simulink model "FCS_MPC_6ph"  (R2022a)
settings: Solver=ode23t  StartTime=0.0  StopTime=0.1  RelTol=1e-3  AbsTol=1e-3  EnableMultiTasking=on
values from neighbouring files (symbols this model uses):
  f_c = 100000    [Params_testbench.m]
  L_d = 0.0001473    [Params_testbench.m]
  L_q = 0.0001484    [Params_testbench.m]
  L_x = 0.00005566    (= 5.566e-05)    [Params_testbench.m]
  L_y = L_x    (= 5.566e-05)    [Params_testbench.m]
  p = 5    [Params_testbench.m]
  psi_pm = 0.0048    [Params_testbench.m]
  R_ph = 0.1278    [Params_testbench.m]
  u_dc = 36.0    (= 36)    [Params_testbench.m]
libraries: nesl_utility x39, fl_lib x32, hdlsllib x25, ee_lib x12, simulink x2, spsAlphaBetaZerotodq0Lib x1
(part 3 of 4)

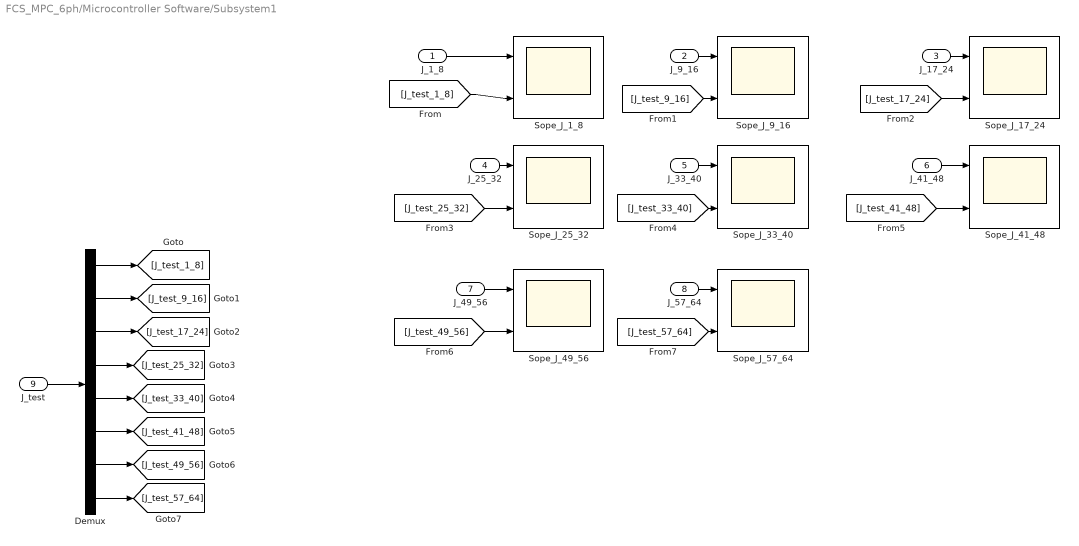
== system FCS_MPC_6ph/Microcontroller Software/Subsystem1 ==
  J_1_8 : Inport
  J_9_16 : Inport  Port=2
  J_17_24 : Inport  Port=3
  J_25_32 : Inport  Port=4
  J_33_40 : Inport  Port=5
  J_41_48 : Inport  Port=6
  J_49_56 : Inport  Port=7
  J_57_64 : Inport  Port=8
  J_test : Inport  Port=9
  Demux : Demux  Outputs=8
  Sope_J_17_24 : Scope  NumInputPorts=2
  Sope_J_1_8 : Scope  NumInputPorts=2
  Sope_J_25_32 : Scope  NumInputPorts=2
  Sope_J_33_40 : Scope  NumInputPorts=2
  Sope_J_41_48 : Scope  NumInputPorts=2
  Sope_J_49_56 : Scope  NumInputPorts=2
  Sope_J_57_64 : Scope  NumInputPorts=2
  Sope_J_9_16 : Scope  NumInputPorts=2
  wires:
  J_test/1 -> Demux/1
  J_1_8/1 -> Sope_J_1_8/1
  Demux/1 -> [J_test_1_8]
  [J_test_1_8] -> Sope_J_1_8/2
  Demux/2 -> [J_test_9_16]
  J_9_16/1 -> Sope_J_9_16/1
  J_17_24/1 -> Sope_J_17_24/1
  J_25_32/1 -> Sope_J_25_32/1
  J_33_40/1 -> Sope_J_33_40/1
  J_41_48/1 -> Sope_J_41_48/1
  J_49_56/1 -> Sope_J_49_56/1
  J_57_64/1 -> Sope_J_57_64/1
  Demux/3 -> [J_test_17_24]
  Demux/4 -> [J_test_25_32]
  Demux/5 -> [J_test_33_40]
  Demux/6 -> [J_test_41_48]
  Demux/7 -> [J_test_49_56]
  Demux/8 -> [J_test_57_64]
  [J_test_9_16] -> Sope_J_9_16/2
  [J_test_17_24] -> Sope_J_17_24/2
  [J_test_25_32] -> Sope_J_25_32/2
  [J_test_33_40] -> Sope_J_33_40/2
  [J_test_41_48] -> Sope_J_41_48/2
  [J_test_49_56] -> Sope_J_49_56/2
  [J_test_57_64] -> Sope_J_57_64/2

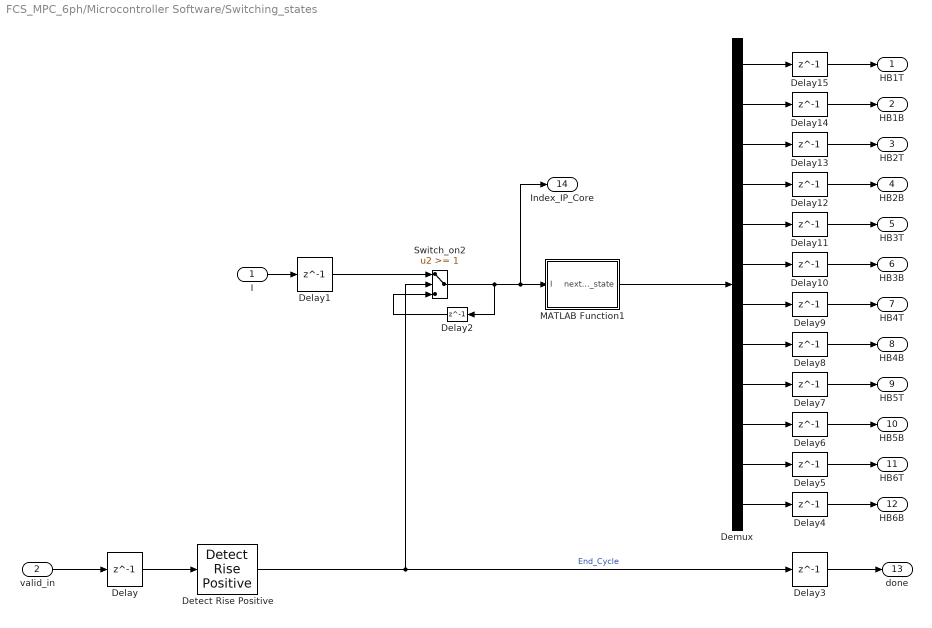
== system FCS_MPC_6ph/Microcontroller Software/Switching_states ==
  I : Inport
  valid_in : Inport  Port=2
  Delay{,1..15} (16 alike) : Delay  DelayLength=1
  Demux : Demux  Outputs=12
  Detect Rise Positive : hdlsllib/Logic and Bit Operations/Detect Rise Positive  vinit=0  OutDataTypeStr=boolean
      settings: SourceProductBaseCode=SL
  MATLAB Function1 : MATLAB Function  TreatAsAtomicUnit=on
  Switch_on2 : Switch  Threshold=1  OutDataTypeStr=Inherit: Inherit via back propagation  RndMeth=Simplest  SaturateOnIntegerOverflow=off  InputSameDT=off
  HB1T : Outport
  HB1B : Outport  Port=2
  HB2T : Outport  Port=3
  HB2B : Outport  Port=4
  HB3T : Outport  Port=5
  HB3B : Outport  Port=6
  HB4T : Outport  Port=7
  HB4B : Outport  Port=8
  HB5T : Outport  Port=9
  HB5B : Outport  Port=10
  HB6T : Outport  Port=11
  HB6B : Outport  Port=12
  done : Outport  Port=13
  Index_IP_Core : Outport  Port=14
  wires:
  Demux/4 -> Delay12/1
  I/1 -> Delay1/1
  Demux/6 -> Delay10/1
  Demux/12 -> Delay4/1
  Demux/8 -> Delay8/1
  valid_in/1 -> Delay/1
  Demux/7 -> Delay9/1
  Demux/2 -> Delay14/1
  Detect Rise Positive/1 -> Delay3/1, Switch_on2/2  "End_Cycle"
  Demux/5 -> Delay11/1
  Delay2/1 -> Switch_on2/3
  Demux/1 -> Delay15/1
  Demux/9 -> Delay7/1
  Demux/10 -> Delay6/1
  MATLAB Function1/1(next_switching_state) -> Demux/1
  Demux/3 -> Delay13/1
  Delay/1 -> Detect Rise Positive/1
  Delay1/1 -> Switch_on2/1
  Delay3/1 -> done/1
  Delay4/1 -> HB6B/1
  Demux/11 -> Delay5/1
  Delay5/1 -> HB6T/1
  Delay6/1 -> HB5B/1
  Delay7/1 -> HB5T/1
  Delay8/1 -> HB4B/1
  Delay9/1 -> HB4T/1
  Delay10/1 -> HB3B/1
  Delay11/1 -> HB3T/1
  Delay12/1 -> HB2B/1
  Delay13/1 -> HB2T/1
  Delay14/1 -> HB1B/1
  Delay15/1 -> HB1T/1
  Switch_on2/1 -> Index_IP_Core/1, MATLAB Function1/1(I), Delay2/1

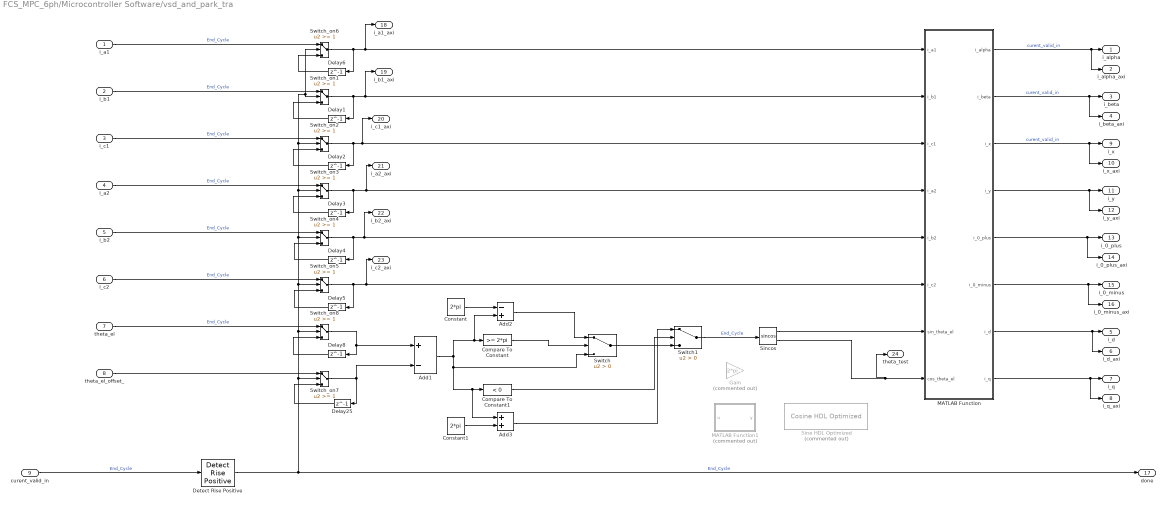
== system FCS_MPC_6ph/Microcontroller Software/vsd_and_park_tra ==
  i_a1 : Inport
  i_b1 : Inport  Port=2
  i_c1 : Inport  Port=3
  i_a2 : Inport  Port=4
  i_b2 : Inport  Port=5
  i_c2 : Inport  Port=6
  theta_el : Inport  Port=7
  theta_el_offset_ : Inport  Port=8
  curent_valid_in : Inport  Port=9
  Add1 : Sum  Inputs=+-  OutDataTypeStr=Inherit: Same as accumulator  RndMeth=Simplest
  Add2 : Sum  Inputs=-+  RndMeth=Simplest  OutDataTypeStr=Inherit: Same as first input
  Add3 : Sum  RndMeth=Simplest  OutDataTypeStr=Inherit: Same as first input
  Compare To Constant : hdlsllib/Logic and Bit Operations/Compare To Constant  relop=>=  const=2*pi  OutDataTypeStr=boolean
      settings: SourceProductBaseCode=SL
  Compare To Constant1 : hdlsllib/Logic and Bit Operations/Compare To Constant  relop=<  const=0  OutDataTypeStr=boolean
      settings: SourceProductBaseCode=SL
  Constant : Constant  Value=2*pi  OutDataTypeStr=single  SampleTime=1.0000e-08
  Constant1 : Constant  Value=2*pi  OutDataTypeStr=single  SampleTime=1.0000e-08
  Delay{1..6,8,25} (8 alike) : Delay  DelayLength=1
  Detect Rise Positive : hdlsllib/Logic and Bit Operations/Detect Rise Positive  vinit=0  OutDataTypeStr=boolean
      settings: SourceProductBaseCode=SL
  Gain : Gain  Commented=on  Gain=2*pi  OutDataTypeStr=Inherit: Same as input  ParamDataTypeStr=Inherit: Same as input
  MATLAB Function : MATLAB Function  TreatAsAtomicUnit=on  SystemSampleTime=1/100000000
  MATLAB Function1 : MATLAB Function  Commented=on  TreatAsAtomicUnit=on
  Sincos : Trigonometry  Operator=sincos
  Sine HDL Optimized : hdlsllib/Lookup Tables/Cosine HDL Optimized  Commented=on  OutputFormula=sin(2*pi*u) and cos(2*pi*u)  NumDataPoints=512  TableDataTypeStr=fixdt(1,17,11)  SimulateLUTROMDelay=off
      settings: SourceProductBaseCode=SL
  Switch : Switch  Criteria=u2 > Threshold  RndMeth=Simplest  SaturateOnIntegerOverflow=off  InputSameDT=off  OutDataTypeStr=Inherit: Same as first input
  Switch1 : Switch  Criteria=u2 > Threshold  RndMeth=Simplest  SaturateOnIntegerOverflow=off  InputSameDT=off  OutDataTypeStr=Inherit: Same as first input
  Switch_on{1..8} (8 alike) : Switch  Threshold=1  RndMeth=Simplest  SaturateOnIntegerOverflow=off  InputSameDT=off  OutDataTypeStr=Inherit: Same as first input
  i_alpha : Outport
  i_alpha_axi : Outport  Port=2
  i_beta : Outport  Port=3
  i_beta_axi : Outport  Port=4
  i_d : Outport  Port=5
  i_d_axi : Outport  Port=6
  i_q : Outport  Port=7
  i_q_axi : Outport  Port=8
  i_x : Outport  Port=9
  i_x_axi : Outport  Port=10
  i_y : Outport  Port=11
  i_y_axi : Outport  Port=12
  i_0_plus : Outport  Port=13
  i_0_plus_axi : Outport  Port=14
  i_0_minus : Outport  Port=15
  i_0_minus_axi : Outport  Port=16
  done : Outport  Port=17
  i_a1_axi : Outport  Port=18
  i_b1_axi : Outport  Port=19
  i_c1_axi : Outport  Port=20
  i_a2_axi : Outport  Port=21
  i_b2_axi : Outport  Port=22
  i_c2_axi : Outport  Port=23
  theta_test : Outport  Port=24
  wires:
  i_c2/1 -> Switch_on5/1  "End_Cycle"
  Switch_on8/1 -> Add1/1, Delay8/1
  Delay8/1 -> Switch_on8/3
  Detect Rise Positive/1 -> done/1, Switch_on7/2, Switch_on6/2, Switch_on1/2, Switch_on2/2, Switch_on3/2, Switch_on4/2, Switch_on5/2, Switch_on8/2  "End_Cycle"
  Delay4/1 -> Switch_on4/3
  Switch_on2/1 -> Delay2/1, i_c1_axi/1, MATLAB Function/3(i_c1)
  Delay1/1 -> Switch_on1/3
  Switch_on1/1 -> Delay1/1, i_b1_axi/1, MATLAB Function/2(i_b1)
  Switch_on6/1 -> i_a1_axi/1, MATLAB Function/1(i_a1), Delay6/1
  Switch_on4/1 -> Delay4/1, i_b2_axi/1, MATLAB Function/5(i_b2)
  curent_valid_in/1 -> Detect Rise Positive/1  "End_Cycle"
  Switch/1 -> Switch1/3
  Switch_on3/1 -> i_a2_axi/1, MATLAB Function/4(i_a2), Delay3/1
  Delay6/1 -> Switch_on6/3
  Constant/1 -> Add2/1
  Add1/1 -> Switch/3, Compare To Constant1/1, Add3/1, Compare To Constant/1, Add2/2
  Delay2/1 -> Switch_on2/3
  Constant1/1 -> Add3/2
  theta_el/1 -> Switch_on8/1  "End_Cycle"
  Delay3/1 -> Switch_on3/3
  i_a1/1 -> Switch_on6/1  "End_Cycle"
  i_b2/1 -> Switch_on4/1  "End_Cycle"
  Add2/1 -> Switch/1
  i_a2/1 -> Switch_on3/1  "End_Cycle"
  i_b1/1 -> Switch_on1/1  "End_Cycle"
  Delay5/1 -> Switch_on5/3
  Add3/1 -> Switch1/1
  i_c1/1 -> Switch_on2/1  "End_Cycle"
  MATLAB Function/1(i_alpha) -> i_alpha_axi/1, i_alpha/1  "curent_valid_in"
  MATLAB Function/2(i_beta) -> i_beta_axi/1, i_beta/1  "curent_valid_in"
  MATLAB Function/3(i_x) -> i_x_axi/1, i_x/1  "curent_valid_in"
  Compare To Constant/1 -> Switch/2
  Compare To Constant1/1 -> Switch1/2
  Switch_on7/1 -> Add1/2, Delay25/1
  Delay25/1 -> Switch_on7/3
  Switch1/1 -> Sincos/1  "End_Cycle"
  ? -> Sine HDL Optimized/1
  theta_el_offset_/1 -> Switch_on7/1
  MATLAB Function/8(i_q) -> i_q_axi/1, i_q/1
  MATLAB Function/7(i_d) -> i_d_axi/1, i_d/1
  MATLAB Function/6(i_0_minus) -> i_0_minus_axi/1, i_0_minus/1
  MATLAB Function/5(i_0_plus) -> i_0_plus_axi/1, i_0_plus/1
  MATLAB Function/4(i_y) -> i_y_axi/1, i_y/1
  Switch_on5/1 -> Delay5/1, i_c2_axi/1, MATLAB Function/6(i_c2)
  Sincos/1 -> MATLAB Function/7(sin_theta_el)
  Sincos/2 -> theta_test/1, MATLAB Function/8(cos_theta_el)

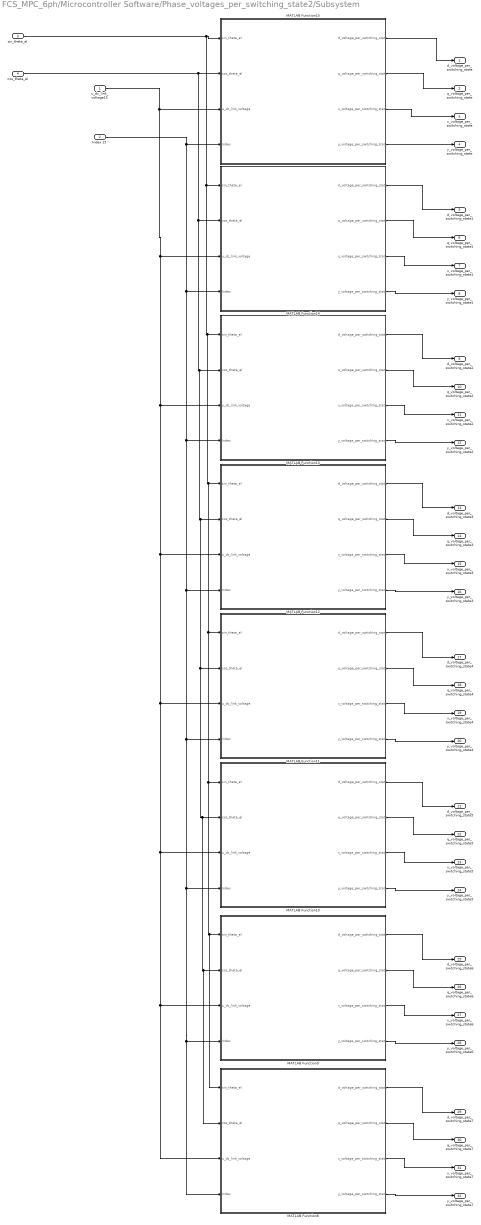
== system FCS_MPC_6ph/Microcontroller Software/Phase_voltages_per_switching_state2/Subsystem ==
  u_dc_link_voltage15 : Inport
  Index 15 : Inport  Port=2
  sin_theta_el : Inport  Port=3
  cos_theta_el : Inport  Port=4
  MATLAB Function10 : MATLAB Function  TreatAsAtomicUnit=on  SystemSampleTime=1/100000000
  MATLAB Function11 : MATLAB Function  TreatAsAtomicUnit=on  SystemSampleTime=1/100000000
  MATLAB Function12 : MATLAB Function  TreatAsAtomicUnit=on  SystemSampleTime=1/100000000
  MATLAB Function13 : MATLAB Function  TreatAsAtomicUnit=on  SystemSampleTime=1/100000000
  MATLAB Function14 : MATLAB Function  TreatAsAtomicUnit=on  SystemSampleTime=1/100000000
  MATLAB Function15 : MATLAB Function  TreatAsAtomicUnit=on  SystemSampleTime=1/100000000
  MATLAB Function8 : MATLAB Function  TreatAsAtomicUnit=on  SystemSampleTime=1/100000000
  MATLAB Function9 : MATLAB Function  TreatAsAtomicUnit=on  SystemSampleTime=1/100000000
  d_voltage_per_switching_state : Outport
  q_voltage_per_switching_state : Outport  Port=2
  x_voltage_per_switching_state : Outport  Port=3
  y_voltage_per_switching_state : Outport  Port=4
  d_voltage_per_switching_state1 : Outport  Port=5
  q_voltage_per_switching_state1 : Outport  Port=6
  x_voltage_per_switching_state1 : Outport  Port=7
  y_voltage_per_switching_state1 : Outport  Port=8
  d_voltage_per_switching_state2 : Outport  Port=9
  q_voltage_per_switching_state2 : Outport  Port=10
  x_voltage_per_switching_state2 : Outport  Port=11
  y_voltage_per_switching_state2 : Outport  Port=12
  d_voltage_per_switching_state3 : Outport  Port=13
  q_voltage_per_switching_state3 : Outport  Port=14
  x_voltage_per_switching_state3 : Outport  Port=15
  y_voltage_per_switching_state3 : Outport  Port=16
  d_voltage_per_switching_state4 : Outport  Port=17
  q_voltage_per_switching_state4 : Outport  Port=18
  x_voltage_per_switching_state4 : Outport  Port=19
  y_voltage_per_switching_state4 : Outport  Port=20
  d_voltage_per_switching_state5 : Outport  Port=21
  q_voltage_per_switching_state5 : Outport  Port=22
  x_voltage_per_switching_state5 : Outport  Port=23
  y_voltage_per_switching_state5 : Outport  Port=24
  d_voltage_per_switching_state6 : Outport  Port=25
  q_voltage_per_switching_state6 : Outport  Port=26
  x_voltage_per_switching_state6 : Outport  Port=27
  y_voltage_per_switching_state6 : Outport  Port=28
  d_voltage_per_switching_state7 : Outport  Port=29
  q_voltage_per_switching_state7 : Outport  Port=30
  x_voltage_per_switching_state7 : Outport  Port=31
  y_voltage_per_switching_state7 : Outport  Port=32
  wires:
  MATLAB Function11/4(y_voltage_per_switching_state) -> y_voltage_per_switching_state4/1
  MATLAB Function10/3(x_voltage_per_switching_state) -> x_voltage_per_switching_state5/1
  MATLAB Function8/1(d_voltage_per_switching_state) -> d_voltage_per_switching_state7/1
  MATLAB Function8/2(q_voltage_per_switching_state) -> q_voltage_per_switching_state7/1
  MATLAB Function11/1(d_voltage_per_switching_state) -> d_voltage_per_switching_state4/1
  MATLAB Function12/3(x_voltage_per_switching_state) -> x_voltage_per_switching_state3/1
  MATLAB Function15/2(q_voltage_per_switching_state) -> q_voltage_per_switching_state/1
  MATLAB Function8/3(x_voltage_per_switching_state) -> x_voltage_per_switching_state7/1
  MATLAB Function11/3(x_voltage_per_switching_state) -> x_voltage_per_switching_state4/1
  MATLAB Function10/4(y_voltage_per_switching_state) -> y_voltage_per_switching_state5/1
  MATLAB Function11/2(q_voltage_per_switching_state) -> q_voltage_per_switching_state4/1
  MATLAB Function12/1(d_voltage_per_switching_state) -> d_voltage_per_switching_state3/1
  MATLAB Function12/4(y_voltage_per_switching_state) -> y_voltage_per_switching_state3/1
  MATLAB Function13/2(q_voltage_per_switching_state) -> q_voltage_per_switching_state2/1
  MATLAB Function10/1(d_voltage_per_switching_state) -> d_voltage_per_switching_state5/1
  MATLAB Function10/2(q_voltage_per_switching_state) -> q_voltage_per_switching_state5/1
  MATLAB Function13/4(y_voltage_per_switching_state) -> y_voltage_per_switching_state2/1
  MATLAB Function8/4(y_voltage_per_switching_state) -> y_voltage_per_switching_state7/1
  MATLAB Function13/1(d_voltage_per_switching_state) -> d_voltage_per_switching_state2/1
  MATLAB Function13/3(x_voltage_per_switching_state) -> x_voltage_per_switching_state2/1
  MATLAB Function12/2(q_voltage_per_switching_state) -> q_voltage_per_switching_state3/1
  MATLAB Function15/1(d_voltage_per_switching_state) -> d_voltage_per_switching_state/1
  MATLAB Function15/4(y_voltage_per_switching_state) -> y_voltage_per_switching_state/1
  MATLAB Function15/3(x_voltage_per_switching_state) -> x_voltage_per_switching_state/1
  u_dc_link_voltage15/1 -> MATLAB Function8/3(u_dc_link_voltage), MATLAB Function9/3(u_dc_link_voltage), MATLAB Function10/3(u_dc_link_voltage), MATLAB Function11/3(u_dc_link_voltage), MATLAB Function12/3(u_dc_link_voltage), MATLAB Function13/3(u_dc_link_voltage), MATLAB Function14/3(u_dc_link_voltage), MATLAB Function15/3(u_dc_link_voltage)
  MATLAB Function14/4(y_voltage_per_switching_state) -> y_voltage_per_switching_state1/1
  MATLAB Function14/3(x_voltage_per_switching_state) -> x_voltage_per_switching_state1/1
  MATLAB Function14/1(d_voltage_per_switching_state) -> d_voltage_per_switching_state1/1
  MATLAB Function14/2(q_voltage_per_switching_state) -> q_voltage_per_switching_state1/1
  Index 15/1 -> MATLAB Function15/4(Index), MATLAB Function10/4(Index), MATLAB Function8/4(Index), MATLAB Function9/4(Index), MATLAB Function11/4(Index), MATLAB Function12/4(Index), MATLAB Function13/4(Index), MATLAB Function14/4(Index)
  MATLAB Function9/3(x_voltage_per_switching_state) -> x_voltage_per_switching_state6/1
  MATLAB Function9/2(q_voltage_per_switching_state) -> q_voltage_per_switching_state6/1
  MATLAB Function9/1(d_voltage_per_switching_state) -> d_voltage_per_switching_state6/1
  MATLAB Function9/4(y_voltage_per_switching_state) -> y_voltage_per_switching_state6/1
  sin_theta_el/1 -> MATLAB Function14/1(sin_theta_el), MATLAB Function8/1(sin_theta_el), MATLAB Function9/1(sin_theta_el), MATLAB Function10/1(sin_theta_el), MATLAB Function11/1(sin_theta_el), MATLAB Function12/1(sin_theta_el), MATLAB Function13/1(sin_theta_el), MATLAB Function15/1(sin_theta_el)
  cos_theta_el/1 -> MATLAB Function15/2(cos_theta_el), MATLAB Function8/2(cos_theta_el), MATLAB Function9/2(cos_theta_el), MATLAB Function10/2(cos_theta_el), MATLAB Function11/2(cos_theta_el), MATLAB Function12/2(cos_theta_el), MATLAB Function13/2(cos_theta_el), MATLAB Function14/2(cos_theta_el)

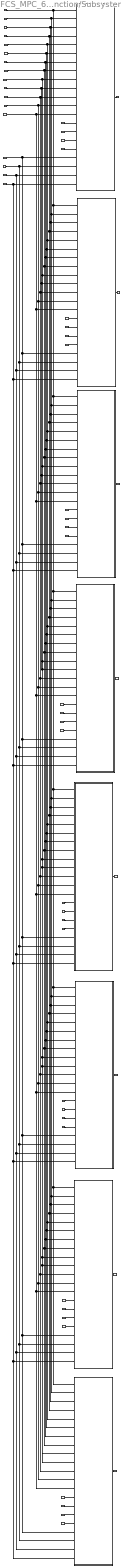
== system FCS_MPC_6ph/Microcontroller Software/Prediction_and_cost_function/Subsystem ==
  d_phase_voltage_per_switching_state : Inport
  q_phase_voltage_per_switching_state : Inport  Port=2
  x_phase_voltage_per_switching_state : Inport  Port=3
  y_phase_voltage_per_switching_state : Inport  Port=4
  d_phase_voltage_per_switching_state1 : Inport  Port=5
  q_phase_voltage_per_switching_state1 : Inport  Port=6
  x_phase_voltage_per_switching_state1 : Inport  Port=7
  y_phase_voltage_per_switching_state1 : Inport  Port=8
  d_phase_voltage_per_switching_state2 : Inport  Port=9
  q_phase_voltage_per_switching_state2 : Inport  Port=10
  x_phase_voltage_per_switching_state2 : Inport  Port=11
  y_phase_voltage_per_switching_state2 : Inport  Port=12
  d_phase_voltage_per_switching_state3 : Inport  Port=13
  q_phase_voltage_per_switching_state3 : Inport  Port=14
  x_phase_voltage_per_switching_state3 : Inport  Port=15
  y_phase_voltage_per_switching_state3 : Inport  Port=16
  d_phase_voltage_per_switching_state4 : Inport  Port=17
  q_phase_voltage_per_switching_state4 : Inport  Port=18
  x_phase_voltage_per_switching_state4 : Inport  Port=19
  y_phase_voltage_per_switching_state4 : Inport  Port=20
  d_phase_voltage_per_switching_state5 : Inport  Port=21
  q_phase_voltage_per_switching_state5 : Inport  Port=22
  x_phase_voltage_per_switching_state5 : Inport  Port=23
  y_phase_voltage_per_switching_state5 : Inport  Port=24
  d_phase_voltage_per_switching_state6 : Inport  Port=25
  q_phase_voltage_per_switching_state6 : Inport  Port=26
  x_phase_voltage_per_switching_state6 : Inport  Port=27
  y_phase_voltage_per_switching_state6 : Inport  Port=28
  d_phase_voltage_per_switching_state7 : Inport  Port=29
  q_phase_voltage_per_switching_state7 : Inport  Port=30
  x_phase_voltage_per_switching_state7 : Inport  Port=31
  y_phase_voltage_per_switching_state7 : Inport  Port=32
  SampleTime_div_Ld15 : Inport  Port=33
  SampleTime_div_Lq15 : Inport  Port=34
  SampleTime_div_Lx15 : Inport  Port=35
  SampleTime_div_Ly15 : Inport  Port=36
  id_k_16 : Inport  Port=37
  iq_k_16 : Inport  Port=38
  ix_k_16 : Inport  Port=39
  iy_k_16 : Inport  Port=40
  Rs15 : Inport  Port=41
  omega_el15 : Inport  Port=42
  Lq15 : Inport  Port=43
  Ld15 : Inport  Port=44
  psiPM15 : Inport  Port=45
  id_ref15 : Inport  Port=46
  iq_ref15 : Inport  Port=47
  ix_ref15 : Inport  Port=48
  iy_ref15 : Inport  Port=49
  MATLAB Function10 : MATLAB Function  TreatAsAtomicUnit=on  SystemSampleTime=1/100000000
  MATLAB Function11 : MATLAB Function  TreatAsAtomicUnit=on  SystemSampleTime=1/100000000
  MATLAB Function12 : MATLAB Function  TreatAsAtomicUnit=on  SystemSampleTime=1/100000000
  MATLAB Function13 : MATLAB Function  TreatAsAtomicUnit=on  SystemSampleTime=1/100000000
  MATLAB Function14 : MATLAB Function  TreatAsAtomicUnit=on  SystemSampleTime=1/100000000
  MATLAB Function15 : MATLAB Function  TreatAsAtomicUnit=on  SystemSampleTime=1/100000000
  MATLAB Function8 : MATLAB Function  TreatAsAtomicUnit=on  SystemSampleTime=1/100000000
  MATLAB Function9 : MATLAB Function  TreatAsAtomicUnit=on  SystemSampleTime=1/100000000
  J : Outport
  J1 : Outport  Port=2
  J2 : Outport  Port=3
  J3 : Outport  Port=4
  J4 : Outport  Port=5
  J5 : Outport  Port=6
  J6 : Outport  Port=7
  J7 : Outport  Port=8
  wires:
  q_phase_voltage_per_switching_state1/1 -> MATLAB Function14/15(q_phase_voltage_per_switching_state)
  SampleTime_div_Ld15/1 -> MATLAB Function8/1(SampleTime_div_Ld), MATLAB Function9/1(SampleTime_div_Ld), MATLAB Function10/1(SampleTime_div_Ld), MATLAB Function11/1(SampleTime_div_Ld), MATLAB Function12/1(SampleTime_div_Ld), MATLAB Function13/1(SampleTime_div_Ld), MATLAB Function14/1(SampleTime_div_Ld), MATLAB Function15/1(SampleTime_div_Ld)
  Rs15/1 -> MATLAB Function8/9(Rs), MATLAB Function9/9(Rs), MATLAB Function10/9(Rs), MATLAB Function11/9(Rs), MATLAB Function12/9(Rs), MATLAB Function13/9(Rs), MATLAB Function14/9(Rs), MATLAB Function15/9(Rs)
  y_phase_voltage_per_switching_state/1 -> MATLAB Function15/17(y_phase_voltage_per_switching_state)
  Lq15/1 -> MATLAB Function8/11(Lq), MATLAB Function9/11(Lq), MATLAB Function10/11(Lq), MATLAB Function11/11(Lq), MATLAB Function12/11(Lq), MATLAB Function13/11(Lq), MATLAB Function14/11(Lq), MATLAB Function15/11(Lq)
  MATLAB Function11/1(J) -> J4/1
  y_phase_voltage_per_switching_state2/1 -> MATLAB Function13/17(y_phase_voltage_per_switching_state)
  d_phase_voltage_per_switching_state1/1 -> MATLAB Function14/14(d_phase_voltage_per_switching_state)
  x_phase_voltage_per_switching_state1/1 -> MATLAB Function14/16(x_phase_voltage_per_switching_state)
  y_phase_voltage_per_switching_state7/1 -> MATLAB Function8/17(y_phase_voltage_per_switching_state)
  iy_ref15/1 -> MATLAB Function8/21(iy_ref), MATLAB Function9/21(iy_ref), MATLAB Function10/21(iy_ref), MATLAB Function11/21(iy_ref), MATLAB Function12/21(iy_ref), MATLAB Function13/21(iy_ref), MATLAB Function14/21(iy_ref), MATLAB Function15/21(iy_ref)
  omega_el15/1 -> MATLAB Function8/10(omega_el), MATLAB Function9/10(omega_el), MATLAB Function10/10(omega_el), MATLAB Function11/10(omega_el), MATLAB Function12/10(omega_el), MATLAB Function13/10(omega_el), MATLAB Function14/10(omega_el), MATLAB Function15/10(omega_el)
  psiPM15/1 -> MATLAB Function8/13(psiPM), MATLAB Function9/13(psiPM), MATLAB Function10/13(psiPM), MATLAB Function11/13(psiPM), MATLAB Function12/13(psiPM), MATLAB Function13/13(psiPM), MATLAB Function14/13(psiPM), MATLAB Function15/13(psiPM)
  d_phase_voltage_per_switching_state3/1 -> MATLAB Function12/14(d_phase_voltage_per_switching_state)
  d_phase_voltage_per_switching_state6/1 -> MATLAB Function9/14(d_phase_voltage_per_switching_state)
  d_phase_voltage_per_switching_state/1 -> MATLAB Function15/14(d_phase_voltage_per_switching_state)
  x_phase_voltage_per_switching_state3/1 -> MATLAB Function12/16(x_phase_voltage_per_switching_state)
  d_phase_voltage_per_switching_state2/1 -> MATLAB Function13/14(d_phase_voltage_per_switching_state)
  x_phase_voltage_per_switching_state4/1 -> MATLAB Function11/16(x_phase_voltage_per_switching_state)
  y_phase_voltage_per_switching_state1/1 -> MATLAB Function14/17(y_phase_voltage_per_switching_state)
  MATLAB Function14/1(J) -> J1/1
  MATLAB Function8/1(J) -> J7/1
  q_phase_voltage_per_switching_state2/1 -> MATLAB Function13/15(q_phase_voltage_per_switching_state)
  x_phase_voltage_per_switching_state2/1 -> MATLAB Function13/16(x_phase_voltage_per_switching_state)
  MATLAB Function13/1(J) -> J2/1
  y_phase_voltage_per_switching_state4/1 -> MATLAB Function11/17(y_phase_voltage_per_switching_state)
  x_phase_voltage_per_switching_state/1 -> MATLAB Function15/16(x_phase_voltage_per_switching_state)
  q_phase_voltage_per_switching_state5/1 -> MATLAB Function10/15(q_phase_voltage_per_switching_state)
  d_phase_voltage_per_switching_state7/1 -> MATLAB Function8/14(d_phase_voltage_per_switching_state)
  d_phase_voltage_per_switching_state4/1 -> MATLAB Function11/14(d_phase_voltage_per_switching_state)
  q_phase_voltage_per_switching_state4/1 -> MATLAB Function11/15(q_phase_voltage_per_switching_state)
  x_phase_voltage_per_switching_state5/1 -> MATLAB Function10/16(x_phase_voltage_per_switching_state)
  SampleTime_div_Lx15/1 -> MATLAB Function8/3(SampleTime_div_Lx), MATLAB Function9/3(SampleTime_div_Lx), MATLAB Function10/3(SampleTime_div_Lx), MATLAB Function11/3(SampleTime_div_Lx), MATLAB Function12/3(SampleTime_div_Lx), MATLAB Function13/3(SampleTime_div_Lx), MATLAB Function14/3(SampleTime_div_Lx), MATLAB Function15/3(SampleTime_div_Lx)
  SampleTime_div_Ly15/1 -> MATLAB Function8/4(SampleTime_div_Ly), MATLAB Function9/4(SampleTime_div_Ly), MATLAB Function10/4(SampleTime_div_Ly), MATLAB Function11/4(SampleTime_div_Ly), MATLAB Function12/4(SampleTime_div_Ly), MATLAB Function13/4(SampleTime_div_Ly), MATLAB Function14/4(SampleTime_div_Ly), MATLAB Function15/4(SampleTime_div_Ly)
  SampleTime_div_Lq15/1 -> MATLAB Function8/2(SampleTime_div_Lq), MATLAB Function9/2(SampleTime_div_Lq), MATLAB Function10/2(SampleTime_div_Lq), MATLAB Function11/2(SampleTime_div_Lq), MATLAB Function12/2(SampleTime_div_Lq), MATLAB Function13/2(SampleTime_div_Lq), MATLAB Function14/2(SampleTime_div_Lq), MATLAB Function15/2(SampleTime_div_Lq)
  x_phase_voltage_per_switching_state7/1 -> MATLAB Function8/16(x_phase_voltage_per_switching_state)
  q_phase_voltage_per_switching_state/1 -> MATLAB Function15/15(q_phase_voltage_per_switching_state)
  MATLAB Function15/1(J) -> J/1
  d_phase_voltage_per_switching_state5/1 -> MATLAB Function10/14(d_phase_voltage_per_switching_state)
  MATLAB Function10/1(J) -> J5/1
  y_phase_voltage_per_switching_state5/1 -> MATLAB Function10/17(y_phase_voltage_per_switching_state)
  q_phase_voltage_per_switching_state6/1 -> MATLAB Function9/15(q_phase_voltage_per_switching_state)
  y_phase_voltage_per_switching_state6/1 -> MATLAB Function9/17(y_phase_voltage_per_switching_state)
  x_phase_voltage_per_switching_state6/1 -> MATLAB Function9/16(x_phase_voltage_per_switching_state)
  MATLAB Function9/1(J) -> J6/1
  MATLAB Function12/1(J) -> J3/1
  q_phase_voltage_per_switching_state7/1 -> MATLAB Function8/15(q_phase_voltage_per_switching_state)
  y_phase_voltage_per_switching_state3/1 -> MATLAB Function12/17(y_phase_voltage_per_switching_state)
  q_phase_voltage_per_switching_state3/1 -> MATLAB Function12/15(q_phase_voltage_per_switching_state)
  ix_ref15/1 -> MATLAB Function8/20(ix_ref), MATLAB Function9/20(ix_ref), MATLAB Function10/20(ix_ref), MATLAB Function11/20(ix_ref), MATLAB Function12/20(ix_ref), MATLAB Function13/20(ix_ref), MATLAB Function14/20(ix_ref), MATLAB Function15/20(ix_ref)
  iq_ref15/1 -> MATLAB Function8/19(iq_ref), MATLAB Function9/19(iq_ref), MATLAB Function10/19(iq_ref), MATLAB Function11/19(iq_ref), MATLAB Function12/19(iq_ref), MATLAB Function13/19(iq_ref), MATLAB Function14/19(iq_ref), MATLAB Function15/19(iq_ref)
  id_ref15/1 -> MATLAB Function8/18(id_ref), MATLAB Function9/18(id_ref), MATLAB Function10/18(id_ref), MATLAB Function11/18(id_ref), MATLAB Function12/18(id_ref), MATLAB Function13/18(id_ref), MATLAB Function14/18(id_ref), MATLAB Function15/18(id_ref)
  Ld15/1 -> MATLAB Function8/12(Ld), MATLAB Function9/12(Ld), MATLAB Function10/12(Ld), MATLAB Function11/12(Ld), MATLAB Function12/12(Ld), MATLAB Function13/12(Ld), MATLAB Function14/12(Ld), MATLAB Function15/12(Ld)
  iy_k_16/1 -> MATLAB Function8/8(iy_k_1), MATLAB Function9/8(iy_k_1), MATLAB Function10/8(iy_k_1), MATLAB Function11/8(iy_k_1), MATLAB Function12/8(iy_k_1), MATLAB Function13/8(iy_k_1), MATLAB Function14/8(iy_k_1), MATLAB Function15/8(iy_k_1)
  ix_k_16/1 -> MATLAB Function8/7(ix_k_1), MATLAB Function9/7(ix_k_1), MATLAB Function10/7(ix_k_1), MATLAB Function11/7(ix_k_1), MATLAB Function12/7(ix_k_1), MATLAB Function13/7(ix_k_1), MATLAB Function14/7(ix_k_1), MATLAB Function15/7(ix_k_1)
  iq_k_16/1 -> MATLAB Function8/6(iq_k_1), MATLAB Function9/6(iq_k_1), MATLAB Function10/6(iq_k_1), MATLAB Function11/6(iq_k_1), MATLAB Function12/6(iq_k_1), MATLAB Function13/6(iq_k_1), MATLAB Function14/6(iq_k_1), MATLAB Function15/6(iq_k_1)
  id_k_16/1 -> MATLAB Function8/5(id_k_1), MATLAB Function9/5(id_k_1), MATLAB Function10/5(id_k_1), MATLAB Function11/5(id_k_1), MATLAB Function12/5(id_k_1), MATLAB Function13/5(id_k_1), MATLAB Function14/5(id_k_1), MATLAB Function15/5(id_k_1)

== matlab function FCS_MPC_6ph/Microcontroller Software/Phase_voltages_per_switching_state2/MATLAB Function1 ==
  settings: fimath=fimath('RoundingMethod', 'Floor','OverflowAction', 'Wrap','ProductMode', 'FullPrecision', 'SumMode', 'FullPrecision')
  data: u input; y output
function y = fcn(u)

    y = fi(u*(1/(2*pi)));

end

== matlab function FCS_MPC_6ph/Microcontroller Software/Switching_states/MATLAB Function1 ==
  data: I input; next_switching_state output
function next_switching_state = fcn(I)

    % Possible switching states of the 6-Phase 2-level inverter
    possible_swichting_states = [0	1	0	1	0	1	0	1	0	1	0	1;
                                1	0	0	1	0	1	0	1	0	1	0	1;
                                0	1	1	0	0	1	0	1	0	1	0	1;
                                1	0	1	0	0	1	0	1	0	1	0	1;
                                0	1	0	1	1	0	0	1	0	1	0	1;
                                1	0	0	1	1	0	0	1	0	1	0	1;
                                0	1	1	0	1	0	0	1	0	1	0	1;
                                1	0	1	0	1	0	0	1	0	1	0	1;
                                0	1	0	1	0	1	1	0	0	1	0	1;
                                1	0	0	1	0	1	1	0	0	1	0	1;
                                0	1	1	0	0	1	1	0	0	1	0	1;
                                1	0	1	0	0	1	1	0	0	1	0	1;
                                0	1	0	1	1	0	1	0	0	1	0	1;
                                1	0	0	1	1	0	1	0	0	1	0	1;
                                0	1	1	0	1	0	1	0	0	1	0	1;
                                1	0	1	0	1	0	1	0	0	1	0	1;
                                0	1	0	1	0	1	0	1	1	0	0	1;
                                1	0	0	1	0	1	0	1	1	0	0	1;
                                0	1	1	0	0	1	0	1	1	0	0	1;
                                1	0	1	0	0	1	0	1	1	0	0	1;
                                0	1	0	1	1	0	0	1	1	0	0	1;
                                1	0	0	1	1	0	0	1	1	0	0	1;
                                0	1	1	0	1	0	0	1	1	0	0	1;
                                1	0	1	0	1	0	0	1	1	0	0	1;
                                0	1	0	1	0	1	1	0	1	0	0	1;
                                1	0	0	1	0	1	1	0	1	0	0	1;
                                0	1	1	0	0	1	1	0	1	0	0	1;
                                1	0	1	0	0	1	1	0	1	0	0	1;
                                0	1	0	1	1	0	1	0	1	0	0	1;
                                1	0	0	1	1	0	1	0	1	0	0	1;
                                0	1	1	0	1	0	1	0	1	0	0	1;
                                1	0	1	0	1	0	1	0	1	0	0	1;
                                0	1	0	1	0	1	0	1	0	1	1	0;
                                1	0	0	1	0	1	0	1	0	1	1	0;
                                0	1	1	0	0	1	0	1	0	1	1	0;
                                1	0	1	0	0	1	0	1	0	1	1	0;
                                0	1	0	1	1	0	0	1	0	1	1	0;
                                1	0	0	1	1	0	0	1	0	1	1	0;
                                0	1	1	0	1	0	0	1	0	1	1	0;
                                1	0	1	0	1	0	0	1	0	1	1	0;
                                0	1	0	1	0	1	1	0	0	1	1	0;
                                1	0	0	1	0	1	1	0	0	1	1	0;
                                0	1	1	0	0	1	1	0	0	1	1	0;
                                1	0	1	0	0	1	1	0	0	1	1	0;
                                0	1	0	1	1	0	1	0	0	1	1	0;
                                1	0	0	1	1	0	1	0	0	1	1	0;
                                0	1	1	0	1	0	1	0	0	1	1	0;
                                1	0	1	0	1	0	1	0	0	1	1	0;
                                0	1	0	1	0	1	0	1	1	0	1	0;
                                1	0	0	1	0	1	0	1	1	0	1	0;
                                0	1	1	0	0	1	0	1	1	0	1	0;
                                1	0	1	0	0	1	0	1	1	0	1	0;
                                0	1	0	1	1	0	0	1	1	0	1	0;
                                1	0	0	1	1	0	0	1	1	0	1	0;
                                0	1	1	0	1	0	0	1	1	0	1	0;
                                1	0	1	0	1	0	0	1	1	0	1	0;
                                0	1	0	1	0	1	1	0	1	0	1	0;
                                1	0	0	1	0	1	1	0	1	0	1	0;
                                0	1	1	0	0	1	1	0	1	0	1	0;
                                1	0	1	0	0	1	1	0	1	0	1	0;
                                0	1	0	1	1	0	1	0	1	0	1	0;
                                1	0	0	1	1	0	1	0	1	0	1	0;
                                0	1	1	0	1	0	1	0	1	0	1	0;
                                1	0	1	0	1	0	1	0	1	0	1	0];

    % Initial condition
    if I==0
        I=int32(1);
    end

    % Output switching state
    next_switching_state=boolean(possible_swichting_states(I,:))';

end

== matlab function FCS_MPC_6ph/6ph_PMSM_30deg_VSD1 ==
  data: u1 input; y1 output; u2 input; u3 input; u4 input; u5 input; u6 input; y2 output; y3 output; y4 output; y5 output; y6 output; k6 input; c6 input
function [y1,y2,y3,y4,y5,y6] = VSD_asymm_30(u1,u2,u3,u4,u5,u6,k6,c6)

A =single([0 0 0 0 0 0]');

A =    k6*[1    -0.5        -0.5        sqrt(3)/2   -sqrt(3)/2  0 ;
           0    sqrt(3)/2   -sqrt(3)/2  0.5         0.5         -1;
           1    -0.5        -0.5        -sqrt(3)/2  sqrt(3)/2   0 ;
           0    -sqrt(3)/2  sqrt(3)/2   0.5         0.5         -1;
           c6   c6          c6          0           0           0 ;
           0    0           0           c6          c6          c6] * [u1 u2 u3 u4 u5 u6]';

y1 =single(A(1));
y2 =single(A(2));
y3 =single(A(3));
y4 =single(A(4));
y5 =single(A(5));
y6 =single(A(6));

== matlab function FCS_MPC_6ph/Microcontroller Software/Prediction_and_cost_function/Subsystem/MATLAB Function8 ==
  data: SampleTime_div_Ld input; J output; SampleTime_div_Lq input; SampleTime_div_Lx input; SampleTime_div_Ly input; id_k_1 input; iq_k_1 input; ix_k_1 input; iy_k_1 input; Rs input; omega_el input; Lq input; Ld input; psiPM input; d_phase_voltage_per_switching_state input; q_phase_voltage_per_switching_state input; x_phase_voltage_per_switching_state input; y_phase_voltage_per_switching_state input; id_ref input; iq_ref input; ix_ref input; iy_ref input
function J = fcn(SampleTime_div_Ld, SampleTime_div_Lq, SampleTime_div_Lx, SampleTime_div_Ly, id_k_1, iq_k_1, ix_k_1, iy_k_1, Rs, omega_el, Lq, Ld, psiPM, d_phase_voltage_per_switching_state, q_phase_voltage_per_switching_state, x_phase_voltage_per_switching_state, y_phase_voltage_per_switching_state, id_ref, iq_ref, ix_ref, iy_ref)
     
        % Prediction of the d-, q-, x-, y-currents of the 6-Phase-PMSM with the finite control set 
        id_k_2 = single(SampleTime_div_Ld*(d_phase_voltage_per_switching_state-id_k_1*Rs+omega_el*Lq*iq_k_1)+id_k_1);
        iq_k_2 = single(SampleTime_div_Lq*(q_phase_voltage_per_switching_state-iq_k_1*Rs-omega_el*(psiPM+id_k_1*Ld))+iq_k_1);
        ix_k_2 = single(SampleTime_div_Lx*(x_phase_voltage_per_switching_state-ix_k_1*Rs)+ix_k_1);
        iy_k_2 = single(SampleTime_div_Ly*(y_phase_voltage_per_switching_state-iy_k_1*Rs)+iy_k_1);
        
        % Calculation of the cost function
        J = single((id_ref-id_k_2)^2+(iq_ref-iq_k_2)^2+(ix_ref-ix_k_2)^2+(iy_ref-iy_k_2)^2);

end

== matlab function FCS_MPC_6ph/Microcontroller Software/Prediction_and_cost_function/Subsystem/MATLAB Function9 ==
  data: SampleTime_div_Ld input; J output; SampleTime_div_Lq input; SampleTime_div_Lx input; SampleTime_div_Ly input; id_k_1 input; iq_k_1 input; ix_k_1 input; iy_k_1 input; Rs input; omega_el input; Lq input; Ld input; psiPM input; d_phase_voltage_per_switching_state input; q_phase_voltage_per_switching_state input; x_phase_voltage_per_switching_state input; y_phase_voltage_per_switching_state input; id_ref input; iq_ref input; ix_ref input; iy_ref input
function J = fcn(SampleTime_div_Ld, SampleTime_div_Lq, SampleTime_div_Lx, SampleTime_div_Ly, id_k_1, iq_k_1, ix_k_1, iy_k_1, Rs, omega_el, Lq, Ld, psiPM, d_phase_voltage_per_switching_state, q_phase_voltage_per_switching_state, x_phase_voltage_per_switching_state, y_phase_voltage_per_switching_state, id_ref, iq_ref, ix_ref, iy_ref)
     
        % Prediction of the d-, q-, x-, y-currents of the 6-Phase-PMSM with the finite control set 
        id_k_2 = single(SampleTime_div_Ld*(d_phase_voltage_per_switching_state-id_k_1*Rs+omega_el*Lq*iq_k_1)+id_k_1);
        iq_k_2 = single(SampleTime_div_Lq*(q_phase_voltage_per_switching_state-iq_k_1*Rs-omega_el*(psiPM+id_k_1*Ld))+iq_k_1);
        ix_k_2 = single(SampleTime_div_Lx*(x_phase_voltage_per_switching_state-ix_k_1*Rs)+ix_k_1);
        iy_k_2 = single(SampleTime_div_Ly*(y_phase_voltage_per_switching_state-iy_k_1*Rs)+iy_k_1);
        
        % Calculation of the cost function
        J = single((id_ref-id_k_2)^2+(iq_ref-iq_k_2)^2+(ix_ref-ix_k_2)^2+(iy_ref-iy_k_2)^2);

end

== matlab function FCS_MPC_6ph/Microcontroller Software/Prediction_and_cost_function/Subsystem/MATLAB Function10 ==
  data: SampleTime_div_Ld input; J output; SampleTime_div_Lq input; SampleTime_div_Lx input; SampleTime_div_Ly input; id_k_1 input; iq_k_1 input; ix_k_1 input; iy_k_1 input; Rs input; omega_el input; Lq input; Ld input; psiPM input; d_phase_voltage_per_switching_state input; q_phase_voltage_per_switching_state input; x_phase_voltage_per_switching_state input; y_phase_voltage_per_switching_state input; id_ref input; iq_ref input; ix_ref input; iy_ref input
function J = fcn(SampleTime_div_Ld, SampleTime_div_Lq, SampleTime_div_Lx, SampleTime_div_Ly, id_k_1, iq_k_1, ix_k_1, iy_k_1, Rs, omega_el, Lq, Ld, psiPM, d_phase_voltage_per_switching_state, q_phase_voltage_per_switching_state, x_phase_voltage_per_switching_state, y_phase_voltage_per_switching_state, id_ref, iq_ref, ix_ref, iy_ref)
     
        % Prediction of the d-, q-, x-, y-currents of the 6-Phase-PMSM with the finite control set 
        id_k_2 = single(SampleTime_div_Ld*(d_phase_voltage_per_switching_state-id_k_1*Rs+omega_el*Lq*iq_k_1)+id_k_1);
        iq_k_2 = single(SampleTime_div_Lq*(q_phase_voltage_per_switching_state-iq_k_1*Rs-omega_el*(psiPM+id_k_1*Ld))+iq_k_1);
        ix_k_2 = single(SampleTime_div_Lx*(x_phase_voltage_per_switching_state-ix_k_1*Rs)+ix_k_1);
        iy_k_2 = single(SampleTime_div_Ly*(y_phase_voltage_per_switching_state-iy_k_1*Rs)+iy_k_1);
        
        % Calculation of the cost function
        J = single((id_ref-id_k_2)^2+(iq_ref-iq_k_2)^2+(ix_ref-ix_k_2)^2+(iy_ref-iy_k_2)^2);

end

== matlab function FCS_MPC_6ph/Microcontroller Software/Prediction_and_cost_function/Subsystem/MATLAB Function11 ==
  data: SampleTime_div_Ld input; J output; SampleTime_div_Lq input; SampleTime_div_Lx input; SampleTime_div_Ly input; id_k_1 input; iq_k_1 input; ix_k_1 input; iy_k_1 input; Rs input; omega_el input; Lq input; Ld input; psiPM input; d_phase_voltage_per_switching_state input; q_phase_voltage_per_switching_state input; x_phase_voltage_per_switching_state input; y_phase_voltage_per_switching_state input; id_ref input; iq_ref input; ix_ref input; iy_ref input
function J = fcn(SampleTime_div_Ld, SampleTime_div_Lq, SampleTime_div_Lx, SampleTime_div_Ly, id_k_1, iq_k_1, ix_k_1, iy_k_1, Rs, omega_el, Lq, Ld, psiPM, d_phase_voltage_per_switching_state, q_phase_voltage_per_switching_state, x_phase_voltage_per_switching_state, y_phase_voltage_per_switching_state, id_ref, iq_ref, ix_ref, iy_ref)
     
        % Prediction of the d-, q-, x-, y-currents of the 6-Phase-PMSM with the finite control set 
        id_k_2 = single(SampleTime_div_Ld*(d_phase_voltage_per_switching_state-id_k_1*Rs+omega_el*Lq*iq_k_1)+id_k_1);
        iq_k_2 = single(SampleTime_div_Lq*(q_phase_voltage_per_switching_state-iq_k_1*Rs-omega_el*(psiPM+id_k_1*Ld))+iq_k_1);
        ix_k_2 = single(SampleTime_div_Lx*(x_phase_voltage_per_switching_state-ix_k_1*Rs)+ix_k_1);
        iy_k_2 = single(SampleTime_div_Ly*(y_phase_voltage_per_switching_state-iy_k_1*Rs)+iy_k_1);
        
        % Calculation of the cost function
        J = single((id_ref-id_k_2)^2+(iq_ref-iq_k_2)^2+(ix_ref-ix_k_2)^2+(iy_ref-iy_k_2)^2);

end

== matlab function FCS_MPC_6ph/Microcontroller Software/Prediction_and_cost_function/Subsystem/MATLAB Function12 ==
  data: SampleTime_div_Ld input; J output; SampleTime_div_Lq input; SampleTime_div_Lx input; SampleTime_div_Ly input; id_k_1 input; iq_k_1 input; ix_k_1 input; iy_k_1 input; Rs input; omega_el input; Lq input; Ld input; psiPM input; d_phase_voltage_per_switching_state input; q_phase_voltage_per_switching_state input; x_phase_voltage_per_switching_state input; y_phase_voltage_per_switching_state input; id_ref input; iq_ref input; ix_ref input; iy_ref input
function J = fcn(SampleTime_div_Ld, SampleTime_div_Lq, SampleTime_div_Lx, SampleTime_div_Ly, id_k_1, iq_k_1, ix_k_1, iy_k_1, Rs, omega_el, Lq, Ld, psiPM, d_phase_voltage_per_switching_state, q_phase_voltage_per_switching_state, x_phase_voltage_per_switching_state, y_phase_voltage_per_switching_state, id_ref, iq_ref, ix_ref, iy_ref)
     
        % Prediction of the d-, q-, x-, y-currents of the 6-Phase-PMSM with the finite control set 
        id_k_2 = single(SampleTime_div_Ld*(d_phase_voltage_per_switching_state-id_k_1*Rs+omega_el*Lq*iq_k_1)+id_k_1);
        iq_k_2 = single(SampleTime_div_Lq*(q_phase_voltage_per_switching_state-iq_k_1*Rs-omega_el*(psiPM+id_k_1*Ld))+iq_k_1);
        ix_k_2 = single(SampleTime_div_Lx*(x_phase_voltage_per_switching_state-ix_k_1*Rs)+ix_k_1);
        iy_k_2 = single(SampleTime_div_Ly*(y_phase_voltage_per_switching_state-iy_k_1*Rs)+iy_k_1);
        
        % Calculation of the cost function
        J = single((id_ref-id_k_2)^2+(iq_ref-iq_k_2)^2+(ix_ref-ix_k_2)^2+(iy_ref-iy_k_2)^2);

end

== matlab function FCS_MPC_6ph/Microcontroller Software/Prediction_and_cost_function/Subsystem/MATLAB Function13 ==
  data: SampleTime_div_Ld input; J output; SampleTime_div_Lq input; SampleTime_div_Lx input; SampleTime_div_Ly input; id_k_1 input; iq_k_1 input; ix_k_1 input; iy_k_1 input; Rs input; omega_el input; Lq input; Ld input; psiPM input; d_phase_voltage_per_switching_state input; q_phase_voltage_per_switching_state input; x_phase_voltage_per_switching_state input; y_phase_voltage_per_switching_state input; id_ref input; iq_ref input; ix_ref input; iy_ref input
function J = fcn(SampleTime_div_Ld, SampleTime_div_Lq, SampleTime_div_Lx, SampleTime_div_Ly, id_k_1, iq_k_1, ix_k_1, iy_k_1, Rs, omega_el, Lq, Ld, psiPM, d_phase_voltage_per_switching_state, q_phase_voltage_per_switching_state, x_phase_voltage_per_switching_state, y_phase_voltage_per_switching_state, id_ref, iq_ref, ix_ref, iy_ref)
     
        % Prediction of the d-, q-, x-, y-currents of the 6-Phase-PMSM with the finite control set 
        id_k_2 = single(SampleTime_div_Ld*(d_phase_voltage_per_switching_state-id_k_1*Rs+omega_el*Lq*iq_k_1)+id_k_1);
        iq_k_2 = single(SampleTime_div_Lq*(q_phase_voltage_per_switching_state-iq_k_1*Rs-omega_el*(psiPM+id_k_1*Ld))+iq_k_1);
        ix_k_2 = single(SampleTime_div_Lx*(x_phase_voltage_per_switching_state-ix_k_1*Rs)+ix_k_1);
        iy_k_2 = single(SampleTime_div_Ly*(y_phase_voltage_per_switching_state-iy_k_1*Rs)+iy_k_1);
        
        % Calculation of the cost function
        J = single((id_ref-id_k_2)^2+(iq_ref-iq_k_2)^2+(ix_ref-ix_k_2)^2+(iy_ref-iy_k_2)^2);

end

== matlab function FCS_MPC_6ph/Microcontroller Software/Prediction_and_cost_function/Subsystem/MATLAB Function14 ==
  data: SampleTime_div_Ld input; J output; SampleTime_div_Lq input; SampleTime_div_Lx input; SampleTime_div_Ly input; id_k_1 input; iq_k_1 input; ix_k_1 input; iy_k_1 input; Rs input; omega_el input; Lq input; Ld input; psiPM input; d_phase_voltage_per_switching_state input; q_phase_voltage_per_switching_state input; x_phase_voltage_per_switching_state input; y_phase_voltage_per_switching_state input; id_ref input; iq_ref input; ix_ref input; iy_ref input
function J = fcn(SampleTime_div_Ld, SampleTime_div_Lq, SampleTime_div_Lx, SampleTime_div_Ly, id_k_1, iq_k_1, ix_k_1, iy_k_1, Rs, omega_el, Lq, Ld, psiPM, d_phase_voltage_per_switching_state, q_phase_voltage_per_switching_state, x_phase_voltage_per_switching_state, y_phase_voltage_per_switching_state, id_ref, iq_ref, ix_ref, iy_ref)
     
        % Prediction of the d-, q-, x-, y-currents of the 6-Phase-PMSM with the finite control set 
        id_k_2 = single(SampleTime_div_Ld*(d_phase_voltage_per_switching_state-id_k_1*Rs+omega_el*Lq*iq_k_1)+id_k_1);
        iq_k_2 = single(SampleTime_div_Lq*(q_phase_voltage_per_switching_state-iq_k_1*Rs-omega_el*(psiPM+id_k_1*Ld))+iq_k_1);
        ix_k_2 = single(SampleTime_div_Lx*(x_phase_voltage_per_switching_state-ix_k_1*Rs)+ix_k_1);
        iy_k_2 = single(SampleTime_div_Ly*(y_phase_voltage_per_switching_state-iy_k_1*Rs)+iy_k_1);
        
        % Calculation of the cost function
        J = single((id_ref-id_k_2)^2+(iq_ref-iq_k_2)^2+(ix_ref-ix_k_2)^2+(iy_ref-iy_k_2)^2);
      

end

== matlab function FCS_MPC_6ph/Microcontroller Software/Prediction_and_cost_function/Subsystem/MATLAB Function15 ==
  data: SampleTime_div_Ld input; J output; SampleTime_div_Lq input; SampleTime_div_Lx input; SampleTime_div_Ly input; id_k_1 input; iq_k_1 input; ix_k_1 input; iy_k_1 input; Rs input; omega_el input; Lq input; Ld input; psiPM input; d_phase_voltage_per_switching_state input; q_phase_voltage_per_switching_state input; x_phase_voltage_per_switching_state input; y_phase_voltage_per_switching_state input; id_ref input; iq_ref input; ix_ref input; iy_ref input
function J = fcn(SampleTime_div_Ld, SampleTime_div_Lq, SampleTime_div_Lx, SampleTime_div_Ly, id_k_1, iq_k_1, ix_k_1, iy_k_1, Rs, omega_el, Lq, Ld, psiPM, d_phase_voltage_per_switching_state, q_phase_voltage_per_switching_state, x_phase_voltage_per_switching_state, y_phase_voltage_per_switching_state, id_ref, iq_ref, ix_ref, iy_ref)
     
        % Prediction of the d-, q-, x-, y-currents of the 6-Phase-PMSM with the finite control set 
        id_k_2 = single(SampleTime_div_Ld*(d_phase_voltage_per_switching_state-id_k_1*Rs+omega_el*Lq*iq_k_1)+id_k_1);
        iq_k_2 = single(SampleTime_div_Lq*(q_phase_voltage_per_switching_state-iq_k_1*Rs-omega_el*(psiPM+id_k_1*Ld))+iq_k_1);
        ix_k_2 = single(SampleTime_div_Lx*(x_phase_voltage_per_switching_state-ix_k_1*Rs)+ix_k_1);
        iy_k_2 = single(SampleTime_div_Ly*(y_phase_voltage_per_switching_state-iy_k_1*Rs)+iy_k_1);
        
        % Calculation of the cost function
        J = single((id_ref-id_k_2)^2+(iq_ref-iq_k_2)^2+(ix_ref-ix_k_2)^2+(iy_ref-iy_k_2)^2);

end

== matlab function FCS_MPC_6ph/Microcontroller Software/Min_cost_function_and_vopt2/MATLAB Function ==
  data: J_1 input single; Index_1 input int32; J output single; voltages_1 input single; J_2 input single; Index_2 input int32; voltages_2 input single; J_3 input single; Index_3 input int32; voltages_3 input single; J_4 input single; Index_4 input int32; voltages_4 input single; J_5 input single; Index_5 input int32; voltages_5 input single; J_6 input single; Index_6 input int32; voltages_6 input single; J_7 input single; Index_7 input int32; voltages_7 input single; J_8 input single; Index_8 input int32; voltages_8 input single; Index output int32; voltages output single; min input single; J_default input single; voltages_default input single
function [J, Index, voltages] = fcn(J_1, Index_1, voltages_1, J_2, Index_2, voltages_2, J_3, Index_3, voltages_3, J_4, Index_4, voltages_4, J_5, Index_5, voltages_5, J_6, Index_6, voltages_6, ...
                                    J_7, Index_7, voltages_7, J_8, Index_8, voltages_8, min, J_default,voltages_default)



if J_1 == min
    Index = Index_1;
    voltages = voltages_1;
    J = J_1;
elseif J_2 == min
    Index = Index_2;
    voltages = voltages_2;
    J = J_2;
elseif J_3 == min
    Index = Index_3;
    voltages = voltages_3;
    J = J_3;
elseif J_4 == min
    Index = Index_4;
    voltages = voltages_4;
    J = J_4;
elseif J_5 == min
    Index = Index_5;
    voltages = voltages_5;
    J = J_5;
elseif J_6 == min
    Index = Index_6;
    voltages = voltages_6;
    J = J_6;
elseif J_7 == min
    Index = Index_7;
    voltages = voltages_7;
    J = J_7;
elseif J_8 == min
    Index = Index_8;
    voltages = voltages_8;
    J = J_8;
else 
    Index = int32(0);
    J = J_default;
    voltages = voltages_default;
end

== matlab function FCS_MPC_6ph/Microcontroller Software/Phase_voltages_per_switching_state2/Subsystem/MATLAB Function10 ==
  data: sin_theta_el input; cos_theta_el input; d_voltage_per_switching_state output; u_dc_link_voltage input; Index input; q_voltage_per_switching_state output; x_voltage_per_switching_state output; y_voltage_per_switching_state output
function [d_voltage_per_switching_state, q_voltage_per_switching_state, x_voltage_per_switching_state, y_voltage_per_switching_state] = fcn(sin_theta_el, cos_theta_el, u_dc_link_voltage, Index)
      
        % Initial condition
            Index = Index+1;

        % Swichtingstates factors alpha beta x y
        Factors_alpha_beta_x_y = single([0.288675134594813	 0.622008467928146	 0.122008467928146	 0.455341801261480    0.122008467928146	 0.455341801261480	-0.0446581987385205  0.288675134594813;
                                         -0.166666666666667	-0.166666666666667	 0.122008467928146	 0.122008467928146   -0.455341801261480	-0.455341801261480	-0.166666666666667	-0.166666666666667;
                                         -0.288675134594813	 0.0446581987385205	-0.455341801261480	-0.122008467928146   -0.455341801261480	-0.122008467928146	-0.622008467928146	-0.288675134594813;
                                         -0.166666666666667	-0.166666666666667	-0.455341801261480	-0.455341801261480    0.122008467928146	 0.122008467928146	-0.166666666666667	-0.166666666666667]);
        
        % Park-Transformation of the switchingstates factors
        Factors_d_q_x_y =single(zeros(4,1));
    
        Factors_d_q_x_y(3,1) = Factors_alpha_beta_x_y(3,Index);
        Factors_d_q_x_y(4,1) = Factors_alpha_beta_x_y(4,Index);
       
        Factors_d_q_x_y(1,1) = cos_theta_el*Factors_alpha_beta_x_y(1,Index)+sin_theta_el*Factors_alpha_beta_x_y(2,Index);
        Factors_d_q_x_y(2,1) = -sin_theta_el*Factors_alpha_beta_x_y(1,Index)+cos_theta_el*Factors_alpha_beta_x_y(2,Index);
    
        %Calculation of the voltages per switching state in alpha beta coordinates
        d_q_x_y_voltages_per_switching_state = single(u_dc_link_voltage*Factors_d_q_x_y);
    
        d_voltage_per_switching_state = d_q_x_y_voltages_per_switching_state(1,1);
        q_voltage_per_switching_state = d_q_x_y_voltages_per_switching_state(2,1);
        x_voltage_per_switching_state = d_q_x_y_voltages_per_switching_state(3,1);
        y_voltage_per_switching_state = d_q_x_y_voltages_per_switching_state(4,1);
    

end
